simulink model "Sim1"  (R2022a)
settings: Solver=FixedStepAuto  StartTime=0.0  StopTime=100  FixedStep=0.01  RelTol=1e-3
values from neighbouring files (symbols this model uses):
  Kd = 0.8    [sim_init.m]
  Kp = 3.5    [sim_init.m]
  q0 = [1,0,-0.3,0]'    [sim_init.m]
settings Model: Creator=ariannagasparri  LastModifiedBy=Marco
settings SolverCC: AlgebraicLoopSolver=TrustRegion
settings DebuggingCC: UnconnectedInputMsg=warning  UnconnectedOutputMsg=warning  UnconnectedLineMsg=warning  SFMachineParentedDataDiag=warning

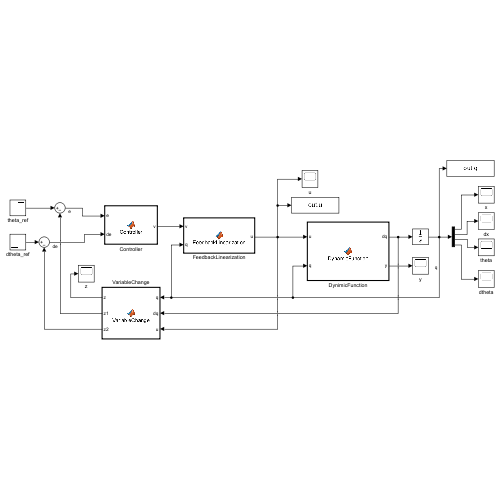
[thumbnail: Simulink's stored preview of the top-level diagram]
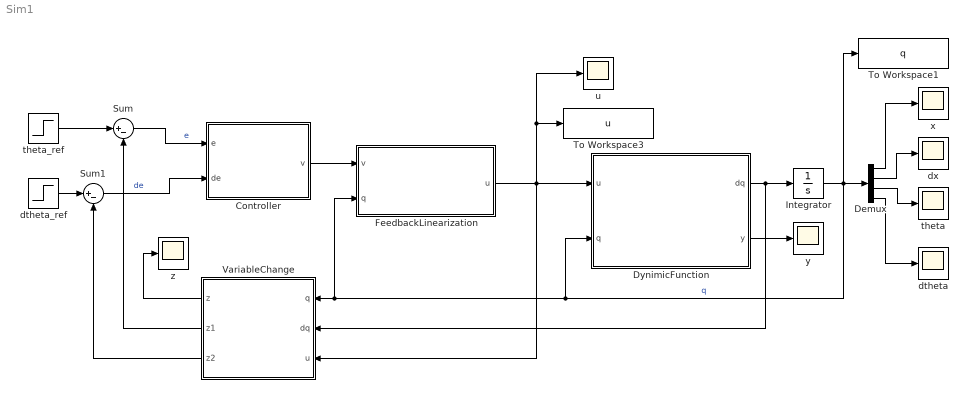
== system Sim1 ==
  Controller : MATLAB Function  TreatAsAtomicUnit=on
  Demux : Demux
  DynimicFunction : MATLAB Function  TreatAsAtomicUnit=on
  FeedbackLinearization : MATLAB Function  TreatAsAtomicUnit=on
  Integrator : Integrator  InitialCondition=q0
  Sum : Sum  Inputs=|+-
  Sum1 : Sum  Inputs=|+-
  To Workspace1 : ToWorkspace  VariableName=q  SaveFormat=Timeseries  SampleTime=-1
  To Workspace3 : ToWorkspace  VariableName=u  SaveFormat=Timeseries  SampleTime=-1
  VariableChange : MATLAB Function  TreatAsAtomicUnit=on
  dtheta : Scope
  dtheta_ref : Step  Time=0  After=0  SampleTime=0
  dx : Scope
  theta : Scope
  theta_ref : Step  Time=0  After=0  SampleTime=0
  u : Scope
  x : Scope
  y : Scope
  z : Scope
  wires:
  DynimicFunction/1(dq) -> Integrator/1, VariableChange/2(dq)
  Sum/1 -> Controller/1(e)  "e"
  Controller/1(v) -> FeedbackLinearization/1(v)
  VariableChange/1(z) -> z/1
  Sum1/1 -> Controller/2(de)  "de"
  Demux/3 -> theta/1
  Demux/1 -> x/1
  Demux/2 -> dx/1
  Integrator/1 -> To Workspace1/1, Demux/1, DynimicFunction/2(q), FeedbackLinearization/2(q), VariableChange/1(q)  "q"
  Demux/4 -> dtheta/1
  dtheta_ref/1 -> Sum1/1
  FeedbackLinearization/1(u) -> u/1, To Workspace3/1, VariableChange/3(u), DynimicFunction/1(u)
  VariableChange/2(z1) -> Sum/2
  VariableChange/3(z2) -> Sum1/2
  theta_ref/1 -> Sum/1
  DynimicFunction/2(y) -> y/1

== matlab function Sim1/FeedbackLinearization ==
  data: v input; u output; q input; param parameter
function u = FeedbackLinearization(v, q, param)

    M = param(1);
    m = param(2);
    l = param(3);
    gravity = param(4);
    b = param(5);
    
    u = ((M+m)*gravity*sin(q(3))+b*q(2)*cos(q(3))-m*l*cos(q(3))*sin(q(3))*q(4)^2)/cos(q(3))-l*v*(M+m*sin(q(3))^2)/cos(q(3)) ;

end

== matlab function Sim1/DynimicFunction ==
  data: u input; dq output; q input; y output; param parameter
function [dq, y] = DynamicFunction(u, q, param)

    M = param(1);
    m = param(2);
    l = param(3);
    gravity = param(4);
    b = param(5);
    
    dq = f_fun(M,b,gravity,l,m,q) + g_fun(M,l,m,q)*u;
    
    y = h_fun(q);

end

== matlab function Sim1/VariableChange ==
  data: q input; dq input; z output; u input; z1 output; z2 output; param parameter
function [z,z1,z2]   = VariableChange(q, dq, u, param)

    z = zeros(4,1);
    dz = zeros(4,1);
    
    M = param(1);
    m = param(2);
    l = param(3);
    gravity = param(4);
    b = param(5);
    
    z(1) = q(3);
    z(2) = q(4);
    z(3) = q(1);
    z(4) = q(2)*cos(q(3)) + l*q(4);
    
    % dz(1) = z(2);
    % dz(2) = dq(1);
    % dz(3) = Lf2h + LgLfh*u; % = v
    % dz(4) = jacobian(z(4),q)*dq;
    
    z1 = z(1);
    z2 = z(2);

end

== matlab function Sim1/Controller ==
  data: e input; de input; v output; Kp parameter; Kd parameter
function v = Controller(e,de, Kp, Kd)

    % Controllo stabilizzante solo angolo
    v = (Kp * e + Kd * de);

end
